simulink model "MALE_UAV_ENGINE"  (R2026a)
settings: Solver=ode45  StopTime=60
(part 1 of 2)
settings Model: Creator=stark  LastModifiedBy=stark
settings DataIOCC: OutputSaveName=simout

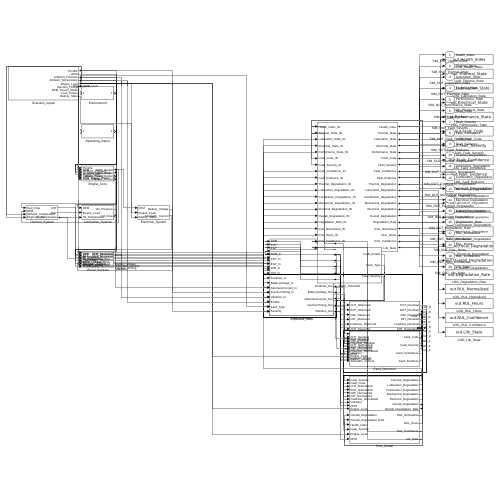
[thumbnail: Simulink's stored preview of the top-level diagram]
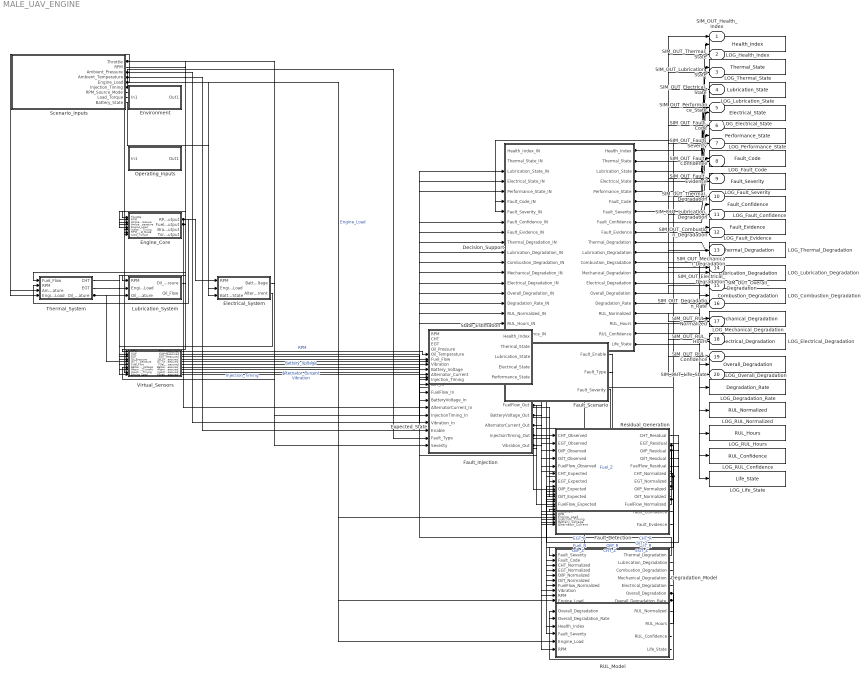
== system MALE_UAV_ENGINE ==
  Decision_Support : Subsystem
  Degradation_Model : Subsystem
  Electrical_System : Subsystem
  Engine_Core : Subsystem
  Environment : Subsystem
  Expected_State : Subsystem
  Fault_Detection : Subsystem
  Fault_Injection : Subsystem
  Fault_Scenario : Subsystem
  LOG_Combustion_Degradation : ToWorkspace  VariableName=Combustion_Degradation  SaveFormat=Timeseries  SampleTime=-1
  LOG_Degradation_Rate : ToWorkspace  VariableName=Degradation_Rate  SaveFormat=Timeseries  SampleTime=-1
  LOG_Electrical_Degradation : ToWorkspace  VariableName=Electrical_Degradation  SaveFormat=Timeseries  SampleTime=-1
  LOG_Electrical_State : ToWorkspace  VariableName=Electrical_State  SaveFormat=Timeseries  SampleTime=-1
  LOG_Fault_Code : ToWorkspace  VariableName=Fault_Code  SaveFormat=Timeseries  SampleTime=-1
  LOG_Fault_Confidence : ToWorkspace  VariableName=Fault_Confidence  SaveFormat=Timeseries  SampleTime=-1
  LOG_Fault_Evidence : ToWorkspace  VariableName=Fault_Evidence  SaveFormat=Timeseries  SampleTime=-1
  LOG_Fault_Severity : ToWorkspace  VariableName=Fault_Severity  SaveFormat=Timeseries  SampleTime=-1
  LOG_Health_Index : ToWorkspace  VariableName=Health_Index  SaveFormat=Timeseries  SampleTime=-1
  LOG_Life_State : ToWorkspace  VariableName=Life_State  SaveFormat=Timeseries  SampleTime=-1
  LOG_Lubrication_Degradation : ToWorkspace  VariableName=Lubrication_Degradation  SaveFormat=Timeseries  SampleTime=-1
  LOG_Lubrication_State : ToWorkspace  VariableName=Lubrication_State  SaveFormat=Timeseries  SampleTime=-1
  LOG_Mechanical_Degradation : ToWorkspace  VariableName=Mechanical_Degradation  SaveFormat=Timeseries  SampleTime=-1
  LOG_Overall_Degradation : ToWorkspace  VariableName=Overall_Degradation  SaveFormat=Timeseries  SampleTime=-1
  LOG_Performance_State : ToWorkspace  VariableName=Performance_State  SaveFormat=Timeseries  SampleTime=-1
  LOG_RUL_Confidence : ToWorkspace  VariableName=RUL_Confidence  SaveFormat=Timeseries  SampleTime=-1
  LOG_RUL_Hours : ToWorkspace  VariableName=RUL_Hours  SaveFormat=Timeseries  SampleTime=-1
  LOG_RUL_Normalized : ToWorkspace  VariableName=RUL_Normalized  SaveFormat=Timeseries  SampleTime=-1
  LOG_Thermal_Degradation : ToWorkspace  VariableName=Thermal_Degradation  SaveFormat=Timeseries  SampleTime=-1
  LOG_Thermal_State : ToWorkspace  VariableName=Thermal_State  SaveFormat=Timeseries  SampleTime=-1
  Lubrication_System : Subsystem
  Operating_Inputs : Subsystem
  RUL_Model : Subsystem
  Residual_Generation : Subsystem
  Scenario_Inputs : Subsystem
  State_Estimation : Subsystem
  Thermal_System : Subsystem
  Virtual_Sensors : Subsystem
  SIM_OUT_Health_Index : Outport  SignalName=Health_Index
  SIM_OUT_Thermal_State : Outport  Port=2  SignalName=Thermal_State
  SIM_OUT_Lubrication_State : Outport  Port=3  SignalName=Lubrication_State
  SIM_OUT_Electrical_State : Outport  Port=4  SignalName=Electrical_State
  SIM_OUT_Performance_State : Outport  Port=5  SignalName=Performance_State
  SIM_OUT_Fault_Code : Outport  Port=6  SignalName=Fault_Code
  SIM_OUT_Fault_Severity : Outport  Port=7  SignalName=Fault_Severity
  SIM_OUT_Fault_Confidence : Outport  Port=8  SignalName=Fault_Confidence
  SIM_OUT_Fault_Evidence : Outport  Port=9  SignalName=Fault_Evidence
  SIM_OUT_Thermal_Degradation : Outport  Port=10  SignalName=Thermal_Degradation
  SIM_OUT_Lubrication_Degradation : Outport  Port=11  SignalName=Lubrication_Degradation
  SIM_OUT_Combustion_Degradation : Outport  Port=12  SignalName=Combustion_Degradation
  SIM_OUT_Mechanical_Degradation : Outport  Port=13  SignalName=Mechanical_Degradation
  SIM_OUT_Electrical_Degradation : Outport  Port=14  SignalName=Electrical_Degradation
  SIM_OUT_Overall_Degradation : Outport  Port=15  SignalName=Overall_Degradation
  SIM_OUT_Degradation_Rate : Outport  Port=16  SignalName=Degradation_Rate
  SIM_OUT_RUL_Normalized : Outport  Port=17  SignalName=RUL_Normalized
  SIM_OUT_RUL_Hours : Outport  Port=18  SignalName=RUL_Hours
  SIM_OUT_RUL_Confidence : Outport  Port=19  SignalName=RUL_Confidence
  SIM_OUT_Life_State : Outport  Port=20  SignalName=Life_State
  wires:
  Scenario_Inputs/1(Throttle) -> Engine_Core/1(Throttle), Expected_State/6(Throttle)
  Scenario_Inputs/2(RPM) -> Engine_Core/2(RPM)
  Scenario_Inputs/3(Ambient_Pressure) -> Engine_Core/3(Ambient_Pressure), Expected_State/3(Ambient_Pressure)
  Scenario_Inputs/4(Ambient_Temperature) -> Engine_Core/4(Ambient_Temperature), Thermal_System/3(Ambient_Temperature), Expected_State/4(Ambient_Temperature)
  Scenario_Inputs/5(Engine_Load) -> Engine_Core/5(Engine_Load), Thermal_System/4(Engine_Load), Lubrication_System/2(Engine_Load), Electrical_System/2(Engine_Load), Virtual_Sensors/10(Engine_Load), Expected_State/2(Engine_Load), Fault_Detection/13(Engine_Load), Degradation_Model/10(Engine_Load), RUL_Model/5(Engine_Load)  "Engine_Load"
  Scenario_Inputs/6(Injection_Timing) -> Engine_Core/6(Injection_Timing), Virtual_Sensors/9(Injection_Timing), Expected_State/5(Injection_Timing)
  Scenario_Inputs/7(RPM_Source_Mode) -> Engine_Core/7(RPM_Source_Mode)
  Scenario_Inputs/8(Load_Torque) -> Engine_Core/8(Load_Torque)
  Engine_Core/2(Fuel_Flow_Output) -> Thermal_System/1(Fuel_Flow), Virtual_Sensors/6(Fuel_Flow)
  Engine_Core/1(RPM_Output) -> Thermal_System/2(RPM), Lubrication_System/1(RPM), Electrical_System/1(RPM), Virtual_Sensors/1(RPM), Expected_State/1(RPM)
  Thermal_System/3(Oil_Temperature) -> Lubrication_System/3(Oil_Temperature), Virtual_Sensors/5(Oil_Temperature)
  Scenario_Inputs/9(Battery_State) -> Electrical_System/3(Battery_State)
  Thermal_System/1(CHT) -> Virtual_Sensors/2(CHT)
  Thermal_System/2(EGT) -> Virtual_Sensors/3(EGT)
  Lubrication_System/1(Oil_Pressure) -> Virtual_Sensors/4(Oil_Pressure)
  Electrical_System/1(Battery_Voltage) -> Virtual_Sensors/7(Battery_Voltage)
  Electrical_System/2(Alternator_Current) -> Virtual_Sensors/8(Alternator_Current)
  Expected_State/1(Expected_CHT) -> Residual_Generation/6(CHT_Expected)
  Expected_State/2(Expected_EGT) -> Residual_Generation/7(EGT_Expected)
  Expected_State/3(Expected_Oil_Pressure) -> Residual_Generation/8(OilP_Expected)
  Expected_State/4(Expected_Oil_Temperature) -> Residual_Generation/9(OilT_Expected)
  Expected_State/5(Expected_Fuel_Flow) -> Residual_Generation/10(FuelFlow_Expected)
  Residual_Generation/1(CHT_Residual) -> Fault_Detection/1(CHT_Residual)  "CHT_R"
  Residual_Generation/2(EGT_Residual) -> Fault_Detection/2(EGT_Residual)  "EGT_R"
  Residual_Generation/3(OilP_Residual) -> Fault_Detection/3(OilP_Residual)  "OilP_R"
  Residual_Generation/4(OilT_Residual) -> Fault_Detection/4(OilT_Residual)  "OilT_R"
  Residual_Generation/5(FuelFlow_Residual) -> Fault_Detection/5(FuelFlow_Residual)  "Fuel_R"
  Residual_Generation/6(CHT_Normalized) -> Fault_Detection/6(CHT_Normalized), Degradation_Model/3(CHT_Normalized)  "CHT_Z"
  Residual_Generation/7(EGT_Normalized) -> Fault_Detection/7(EGT_Normalized), Degradation_Model/4(EGT_Normalized)  "EGT_Z"
  Residual_Generation/8(OilP_Normalized) -> Fault_Detection/8(OilP_Normalized), Degradation_Model/5(OilP_Normalized)  "OilP_Z"
  Residual_Generation/9(OilT_Normalized) -> Fault_Detection/9(OilT_Normalized), Degradation_Model/6(OilT_Normalized)  "OilT_Z"
  Residual_Generation/10(FuelFlow_Normalized) -> Fault_Detection/10(FuelFlow_Normalized), Degradation_Model/7(FuelFlow_Normalized)  "Fuel_Z"
  Fault_Detection/2(Fault_Severity) -> Degradation_Model/1(Fault_Severity), RUL_Model/4(Fault_Severity), Decision_Support/7(Fault_Severity_IN)
  Fault_Detection/1(Fault_Code) -> Degradation_Model/2(Fault_Code), Decision_Support/6(Fault_Code_IN)
  Degradation_Model/6(Overall_Degradation) -> RUL_Model/1(Overall_Degradation), Decision_Support/15(Overall_Degradation_IN)
  Degradation_Model/7(Overall_Degradation_Rate) -> RUL_Model/2(Overall_Degradation_Rate), Decision_Support/16(Degradation_Rate_IN)
  State_Estimation/1(Health_Index) -> RUL_Model/3(Health_Index), Decision_Support/1(Health_Index_IN)
  State_Estimation/2(Thermal_State) -> Decision_Support/2(Thermal_State_IN)
  State_Estimation/3(Lubrication_State) -> Decision_Support/3(Lubrication_State_IN)
  State_Estimation/4(Electrical_State) -> Decision_Support/4(Electrical_State_IN)
  State_Estimation/5(Performance_State) -> Decision_Support/5(Performance_State_IN)
  Fault_Detection/3(Fault_Confidence) -> Decision_Support/8(Fault_Confidence_IN)
  Fault_Detection/4(Fault_Evidence) -> Decision_Support/9(Fault_Evidence_IN)
  Degradation_Model/1(Thermal_Degradation) -> Decision_Support/10(Thermal_Degradation_IN)
  Degradation_Model/2(Lubrication_Degradation) -> Decision_Support/11(Lubrication_Degradation_IN)
  Degradation_Model/3(Combustion_Degradation) -> Decision_Support/12(Combustion_Degradation_IN)
  Degradation_Model/4(Mechanical_Degradation) -> Decision_Support/13(Mechanical_Degradation_IN)
  Degradation_Model/5(Electrical_Degradation) -> Decision_Support/14(Electrical_Degradation_IN)
  RUL_Model/1(RUL_Normalized) -> Decision_Support/17(RUL_Normalized_IN)
  RUL_Model/2(RUL_Hours) -> Decision_Support/18(RUL_Hours_IN)
  RUL_Model/3(RUL_Confidence) -> Decision_Support/19(RUL_Confidence_IN)
  RUL_Model/4(Life_State) -> Decision_Support/20(Life_State_IN)
  Decision_Support/1(Health_Index) -> LOG_Health_Index/1, SIM_OUT_Health_Index/1
  Decision_Support/2(Thermal_State) -> LOG_Thermal_State/1, SIM_OUT_Thermal_State/1
  Decision_Support/3(Lubrication_State) -> LOG_Lubrication_State/1, SIM_OUT_Lubrication_State/1
  Decision_Support/4(Electrical_State) -> LOG_Electrical_State/1, SIM_OUT_Electrical_State/1
  Decision_Support/5(Performance_State) -> LOG_Performance_State/1, SIM_OUT_Performance_State/1
  Decision_Support/6(Fault_Code) -> LOG_Fault_Code/1, SIM_OUT_Fault_Code/1
  Decision_Support/7(Fault_Severity) -> LOG_Fault_Severity/1, SIM_OUT_Fault_Severity/1
  Decision_Support/8(Fault_Confidence) -> LOG_Fault_Confidence/1, SIM_OUT_Fault_Confidence/1
  Decision_Support/9(Fault_Evidence) -> LOG_Fault_Evidence/1, SIM_OUT_Fault_Evidence/1
  Decision_Support/10(Thermal_Degradation) -> LOG_Thermal_Degradation/1, SIM_OUT_Thermal_Degradation/1
  Decision_Support/11(Lubrication_Degradation) -> LOG_Lubrication_Degradation/1, SIM_OUT_Lubrication_Degradation/1
  Decision_Support/12(Combustion_Degradation) -> LOG_Combustion_Degradation/1, SIM_OUT_Combustion_Degradation/1
  Decision_Support/13(Mechanical_Degradation) -> LOG_Mechanical_Degradation/1, SIM_OUT_Mechanical_Degradation/1
  Decision_Support/14(Electrical_Degradation) -> LOG_Electrical_Degradation/1, SIM_OUT_Electrical_Degradation/1
  Decision_Support/15(Overall_Degradation) -> LOG_Overall_Degradation/1, SIM_OUT_Overall_Degradation/1
  Decision_Support/16(Degradation_Rate) -> LOG_Degradation_Rate/1, SIM_OUT_Degradation_Rate/1
  Decision_Support/17(RUL_Normalized) -> LOG_RUL_Normalized/1, SIM_OUT_RUL_Normalized/1
  Decision_Support/18(RUL_Hours) -> LOG_RUL_Hours/1, SIM_OUT_RUL_Hours/1
  Decision_Support/19(RUL_Confidence) -> LOG_RUL_Confidence/1, SIM_OUT_RUL_Confidence/1
  Decision_Support/20(Life_State) -> LOG_Life_State/1, SIM_OUT_Life_State/1
  Fault_Scenario/1(Fault_Enable) -> Fault_Injection/11(Enable)
  Fault_Scenario/2(Fault_Type) -> Fault_Injection/12(Fault_Type)
  Fault_Scenario/3(Fault_Severity) -> Fault_Injection/13(Severity)
  Virtual_Sensors/1(RPM_Measured) -> Fault_Injection/1(RPM_In)  "RPM"
  Virtual_Sensors/2(CHT_Measured) -> Fault_Injection/2(CHT_In)
  Virtual_Sensors/3(EGT_Measured) -> Fault_Injection/3(EGT_In)
  Virtual_Sensors/4(Oil_Pressure_Measured) -> Fault_Injection/4(OilP_In)
  Virtual_Sensors/5(Oil_Temperature_Measured) -> Fault_Injection/5(OilT_In)
  Virtual_Sensors/6(Fuel_Flow_Measured) -> Fault_Injection/6(FuelFlow_In)
  Virtual_Sensors/7(Battery_Voltage_Measured) -> Fault_Injection/7(BatteryVoltage_In)  "Battery_Voltage"
  Virtual_Sensors/8(Alternator_Current_Measured) -> Fault_Injection/8(AlternatorCurrent_In)  "Alternator_Current"
  Virtual_Sensors/9(Injection_Timing_Measured) -> Fault_Injection/9(InjectionTiming_In)  "Injection_Timing"
  Virtual_Sensors/10(Vibration_Measured) -> Fault_Injection/10(Vibration_In)  "Vibration"
  Fault_Injection/1(RPM_Out) -> State_Estimation/1(RPM), Fault_Detection/12(RPM), Degradation_Model/9(RPM), RUL_Model/6(RPM)
  Fault_Injection/2(CHT_Out) -> State_Estimation/2(CHT), Residual_Generation/1(CHT_Observed)
  Fault_Injection/3(EGT_Out) -> State_Estimation/3(EGT), Residual_Generation/2(EGT_Observed)
  Fault_Injection/4(OilP_Out) -> State_Estimation/4(Oil_Pressure), Residual_Generation/3(OilP_Observed)
  Fault_Injection/5(OilT_Out) -> State_Estimation/5(Oil_Temperature), Residual_Generation/4(OilT_Observed)
  Fault_Injection/6(FuelFlow_Out) -> State_Estimation/6(Fuel_Flow), Residual_Generation/5(FuelFlow_Observed)
  Fault_Injection/7(BatteryVoltage_Out) -> State_Estimation/8(Battery_Voltage), Fault_Detection/15(Battery_Voltage)
  Fault_Injection/8(AlternatorCurrent_Out) -> State_Estimation/9(Alternator_Current), Fault_Detection/16(Alternator_Current)
  Fault_Injection/9(InjectionTiming_Out) -> State_Estimation/10(Injection_Timing), Fault_Detection/14(Injection_Timing)
  Fault_Injection/10(Vibration_Out) -> State_Estimation/7(Vibration), Fault_Detection/11(Vibration), Degradation_Model/8(Vibration)

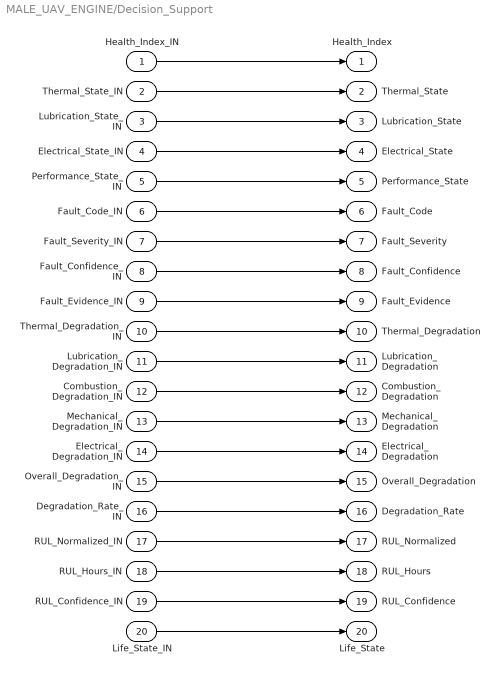
== system MALE_UAV_ENGINE/Decision_Support ==
  Health_Index_IN : Inport
  Thermal_State_IN : Inport  Port=2
  Lubrication_State_IN : Inport  Port=3
  Electrical_State_IN : Inport  Port=4
  Performance_State_IN : Inport  Port=5
  Fault_Code_IN : Inport  Port=6
  Fault_Severity_IN : Inport  Port=7
  Fault_Confidence_IN : Inport  Port=8
  Fault_Evidence_IN : Inport  Port=9
  Thermal_Degradation_IN : Inport  Port=10
  Lubrication_Degradation_IN : Inport  Port=11
  Combustion_Degradation_IN : Inport  Port=12
  Mechanical_Degradation_IN : Inport  Port=13
  Electrical_Degradation_IN : Inport  Port=14
  Overall_Degradation_IN : Inport  Port=15
  Degradation_Rate_IN : Inport  Port=16
  RUL_Normalized_IN : Inport  Port=17
  RUL_Hours_IN : Inport  Port=18
  RUL_Confidence_IN : Inport  Port=19
  Life_State_IN : Inport  Port=20
  Health_Index : Outport
  Thermal_State : Outport  Port=2
  Lubrication_State : Outport  Port=3
  Electrical_State : Outport  Port=4
  Performance_State : Outport  Port=5
  Fault_Code : Outport  Port=6
  Fault_Severity : Outport  Port=7
  Fault_Confidence : Outport  Port=8
  Fault_Evidence : Outport  Port=9
  Thermal_Degradation : Outport  Port=10
  Lubrication_Degradation : Outport  Port=11
  Combustion_Degradation : Outport  Port=12
  Mechanical_Degradation : Outport  Port=13
  Electrical_Degradation : Outport  Port=14
  Overall_Degradation : Outport  Port=15
  Degradation_Rate : Outport  Port=16
  RUL_Normalized : Outport  Port=17
  RUL_Hours : Outport  Port=18
  RUL_Confidence : Outport  Port=19
  Life_State : Outport  Port=20
  wires:
  ? -> ?
  Health_Index_IN/1 -> Health_Index/1
  Thermal_State_IN/1 -> Thermal_State/1
  Lubrication_State_IN/1 -> Lubrication_State/1
  Electrical_State_IN/1 -> Electrical_State/1
  Performance_State_IN/1 -> Performance_State/1
  Fault_Code_IN/1 -> Fault_Code/1
  Fault_Severity_IN/1 -> Fault_Severity/1
  Fault_Confidence_IN/1 -> Fault_Confidence/1
  Fault_Evidence_IN/1 -> Fault_Evidence/1
  Thermal_Degradation_IN/1 -> Thermal_Degradation/1
  Lubrication_Degradation_IN/1 -> Lubrication_Degradation/1
  Combustion_Degradation_IN/1 -> Combustion_Degradation/1
  Mechanical_Degradation_IN/1 -> Mechanical_Degradation/1
  Electrical_Degradation_IN/1 -> Electrical_Degradation/1
  Overall_Degradation_IN/1 -> Overall_Degradation/1
  Degradation_Rate_IN/1 -> Degradation_Rate/1
  RUL_Normalized_IN/1 -> RUL_Normalized/1
  RUL_Hours_IN/1 -> RUL_Hours/1
  RUL_Confidence_IN/1 -> RUL_Confidence/1
  Life_State_IN/1 -> Life_State/1

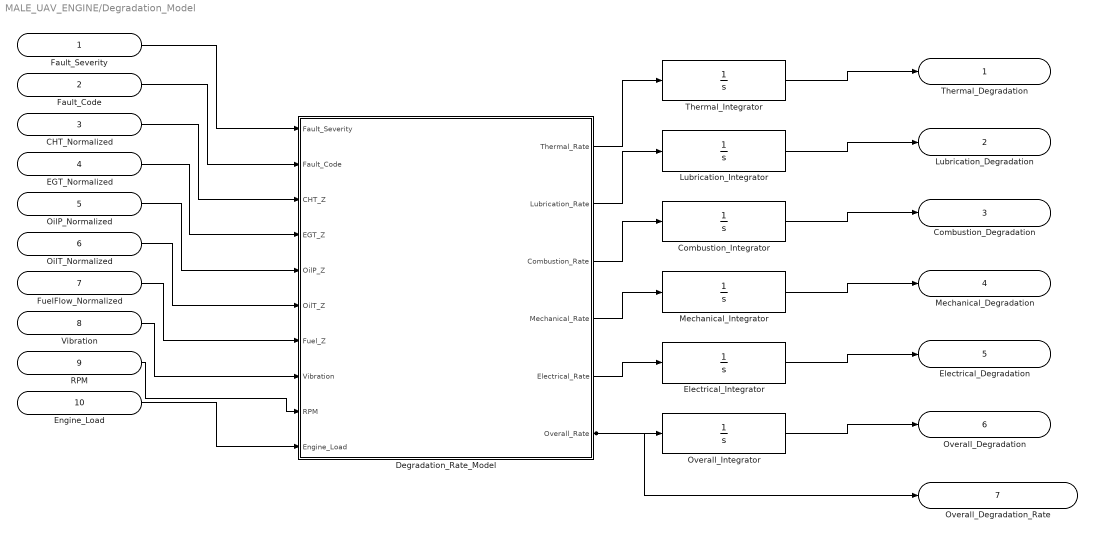
== system MALE_UAV_ENGINE/Degradation_Model ==
  Fault_Severity : Inport
  Fault_Code : Inport  Port=2
  CHT_Normalized : Inport  Port=3
  EGT_Normalized : Inport  Port=4
  OilP_Normalized : Inport  Port=5
  OilT_Normalized : Inport  Port=6
  FuelFlow_Normalized : Inport  Port=7
  Vibration : Inport  Port=8
  RPM : Inport  Port=9
  Engine_Load : Inport  Port=10
  Combustion_Integrator : Integrator  LimitOutput=on  UpperSaturationLimit=1  LowerSaturationLimit=0
  Degradation_Rate_Model : MATLAB Function  TreatAsAtomicUnit=on
  Electrical_Integrator : Integrator  LimitOutput=on  UpperSaturationLimit=1  LowerSaturationLimit=0
  Lubrication_Integrator : Integrator  LimitOutput=on  UpperSaturationLimit=1  LowerSaturationLimit=0
  Mechanical_Integrator : Integrator  LimitOutput=on  UpperSaturationLimit=1  LowerSaturationLimit=0
  Overall_Integrator : Integrator  LimitOutput=on  UpperSaturationLimit=1  LowerSaturationLimit=0
  Thermal_Integrator : Integrator  LimitOutput=on  UpperSaturationLimit=1  LowerSaturationLimit=0
  Thermal_Degradation : Outport
  Lubrication_Degradation : Outport  Port=2
  Combustion_Degradation : Outport  Port=3
  Mechanical_Degradation : Outport  Port=4
  Electrical_Degradation : Outport  Port=5
  Overall_Degradation : Outport  Port=6
  Overall_Degradation_Rate : Outport  Port=7
  wires:
  Fault_Severity/1 -> Degradation_Rate_Model/1(Fault_Severity)
  Fault_Code/1 -> Degradation_Rate_Model/2(Fault_Code)
  CHT_Normalized/1 -> Degradation_Rate_Model/3(CHT_Z)
  EGT_Normalized/1 -> Degradation_Rate_Model/4(EGT_Z)
  OilP_Normalized/1 -> Degradation_Rate_Model/5(OilP_Z)
  OilT_Normalized/1 -> Degradation_Rate_Model/6(OilT_Z)
  FuelFlow_Normalized/1 -> Degradation_Rate_Model/7(Fuel_Z)
  Vibration/1 -> Degradation_Rate_Model/8(Vibration)
  RPM/1 -> Degradation_Rate_Model/9(RPM)
  Engine_Load/1 -> Degradation_Rate_Model/10(Engine_Load)
  Degradation_Rate_Model/1(Thermal_Rate) -> Thermal_Integrator/1
  Degradation_Rate_Model/2(Lubrication_Rate) -> Lubrication_Integrator/1
  Degradation_Rate_Model/3(Combustion_Rate) -> Combustion_Integrator/1
  Degradation_Rate_Model/4(Mechanical_Rate) -> Mechanical_Integrator/1
  Degradation_Rate_Model/5(Electrical_Rate) -> Electrical_Integrator/1
  Degradation_Rate_Model/6(Overall_Rate) -> Overall_Integrator/1, Overall_Degradation_Rate/1
  Thermal_Integrator/1 -> Thermal_Degradation/1
  Lubrication_Integrator/1 -> Lubrication_Degradation/1
  Combustion_Integrator/1 -> Combustion_Degradation/1
  Mechanical_Integrator/1 -> Mechanical_Degradation/1
  Electrical_Integrator/1 -> Electrical_Degradation/1
  Overall_Integrator/1 -> Overall_Degradation/1

== system MALE_UAV_ENGINE/Electrical_System ==
  RPM : Inport
  Engine_Load : Inport  Port=2
  Battery_State : Inport  Port=3
  Battery_Voltage_Dynamics : TransferFcn  Denominator=[0.8 1]
  Electrical_Model : MATLAB Function  TreatAsAtomicUnit=on
  Battery_Voltage : Outport
  Alternator_Current : Outport  Port=2
  wires:
  RPM/1 -> Electrical_Model/1(RPM)
  Engine_Load/1 -> Electrical_Model/2(Engine_Load)
  Battery_State/1 -> Electrical_Model/3(Battery_State)
  Electrical_Model/1(Battery_Voltage) -> Battery_Voltage_Dynamics/1
  Battery_Voltage_Dynamics/1 -> Battery_Voltage/1
  Electrical_Model/2(Alternator_Current) -> Alternator_Current/1

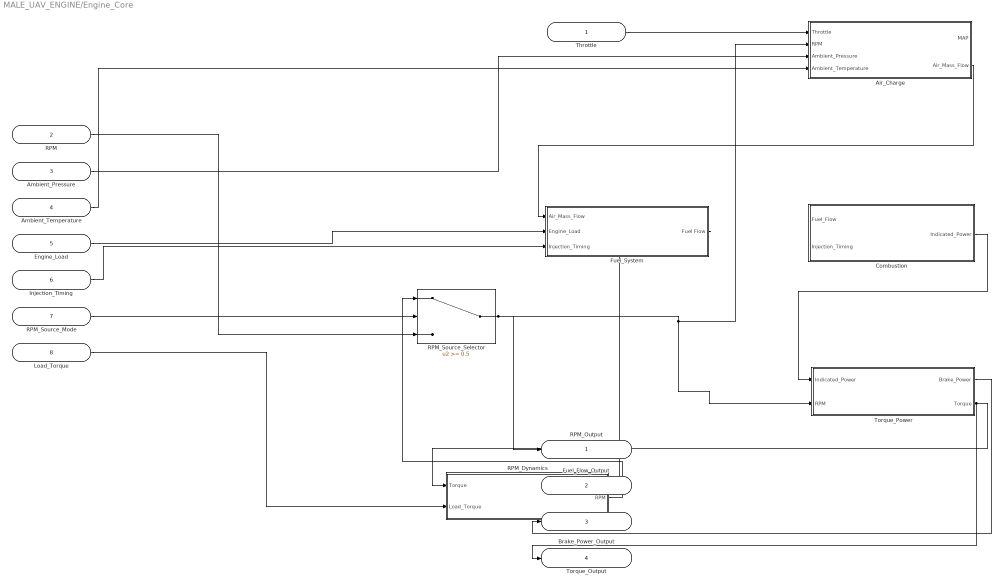
== system MALE_UAV_ENGINE/Engine_Core ==
  Throttle : Inport
  RPM : Inport  Port=2
  Ambient_Pressure : Inport  Port=3
  Ambient_Temperature : Inport  Port=4
  Engine_Load : Inport  Port=5
  Injection_Timing : Inport  Port=6
  RPM_Source_Mode : Inport  Port=7
  Load_Torque : Inport  Port=8
  Air_Charge : Subsystem
  Combustion : Subsystem
  Fuel_System : Subsystem
  RPM_Dynamics : Subsystem
  RPM_Source_Selector : Switch  Threshold=0.5  SaturateOnIntegerOverflow=off  InputSameDT=off
  Torque_Power : Subsystem
  RPM_Output : Outport
  Fuel_Flow_Output : Outport  Port=2
  Brake_Power_Output : Outport  Port=3
  Torque_Output : Outport  Port=4
  wires:
  Throttle/1 -> Air_Charge/1(Throttle)
  Ambient_Pressure/1 -> Air_Charge/3(Ambient_Pressure)
  Ambient_Temperature/1 -> Air_Charge/4(Ambient_Temperature)
  Engine_Load/1 -> Fuel_System/2(Engine_Load)
  Injection_Timing/1 -> Fuel_System/3(Injection_Timing)
  Air_Charge/2(Air_Mass_Flow) -> Fuel_System/1(Air_Mass_Flow)
  RPM_Dynamics/1(RPM) -> RPM_Source_Selector/1
  RPM_Source_Mode/1 -> RPM_Source_Selector/2
  RPM/1 -> RPM_Source_Selector/3
  RPM_Source_Selector/1 -> Torque_Power/2(RPM), Air_Charge/2(RPM), RPM_Output/1
  Combustion/1(Indicated_Power) -> Torque_Power/1(Indicated_Power)
  Torque_Power/2(Torque) -> RPM_Dynamics/1(Torque), Torque_Output/1
  Load_Torque/1 -> RPM_Dynamics/2(Load_Torque)
  Fuel_System/1(Fuel Flow) -> Fuel_Flow_Output/1
  Torque_Power/1(Brake_Power) -> Brake_Power_Output/1

== system MALE_UAV_ENGINE/Environment ==
  In1 : Inport
  Out1 : Outport
  wires:
  In1/1 -> Out1/1

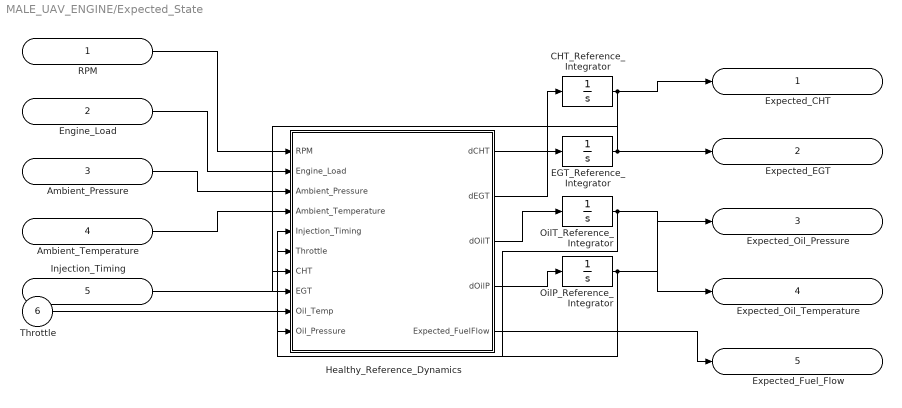
== system MALE_UAV_ENGINE/Expected_State ==
  RPM : Inport
  Engine_Load : Inport  Port=2
  Ambient_Pressure : Inport  Port=3
  Ambient_Temperature : Inport  Port=4
  Injection_Timing : Inport  Port=5
  Throttle : Inport  Port=6
  CHT_Reference_Integrator : Integrator  InitialCondition=373.15
  EGT_Reference_Integrator : Integrator  InitialCondition=873.15
  Healthy_Reference_Dynamics : MATLAB Function  TreatAsAtomicUnit=on
  OilP_Reference_Integrator : Integrator
  OilT_Reference_Integrator : Integrator  InitialCondition=363.15
  Expected_CHT : Outport
  Expected_EGT : Outport  Port=2
  Expected_Oil_Pressure : Outport  Port=3
  Expected_Oil_Temperature : Outport  Port=4
  Expected_Fuel_Flow : Outport  Port=5
  wires:
  RPM/1 -> Healthy_Reference_Dynamics/1(RPM)
  Engine_Load/1 -> Healthy_Reference_Dynamics/2(Engine_Load)
  Ambient_Pressure/1 -> Healthy_Reference_Dynamics/3(Ambient_Pressure)
  Ambient_Temperature/1 -> Healthy_Reference_Dynamics/4(Ambient_Temperature)
  Injection_Timing/1 -> Healthy_Reference_Dynamics/5(Injection_Timing)
  Throttle/1 -> Healthy_Reference_Dynamics/6(Throttle)
  CHT_Reference_Integrator/1 -> Healthy_Reference_Dynamics/7(CHT), Expected_CHT/1
  EGT_Reference_Integrator/1 -> Healthy_Reference_Dynamics/8(EGT), Expected_EGT/1
  OilT_Reference_Integrator/1 -> Healthy_Reference_Dynamics/9(Oil_Temp), Expected_Oil_Temperature/1
  OilP_Reference_Integrator/1 -> Healthy_Reference_Dynamics/10(Oil_Pressure), Expected_Oil_Pressure/1
  Healthy_Reference_Dynamics/1(dCHT) -> CHT_Reference_Integrator/1
  Healthy_Reference_Dynamics/2(dEGT) -> EGT_Reference_Integrator/1
  Healthy_Reference_Dynamics/3(dOilT) -> OilT_Reference_Integrator/1
  Healthy_Reference_Dynamics/4(dOilP) -> OilP_Reference_Integrator/1
  Healthy_Reference_Dynamics/5(Expected_FuelFlow) -> Expected_Fuel_Flow/1

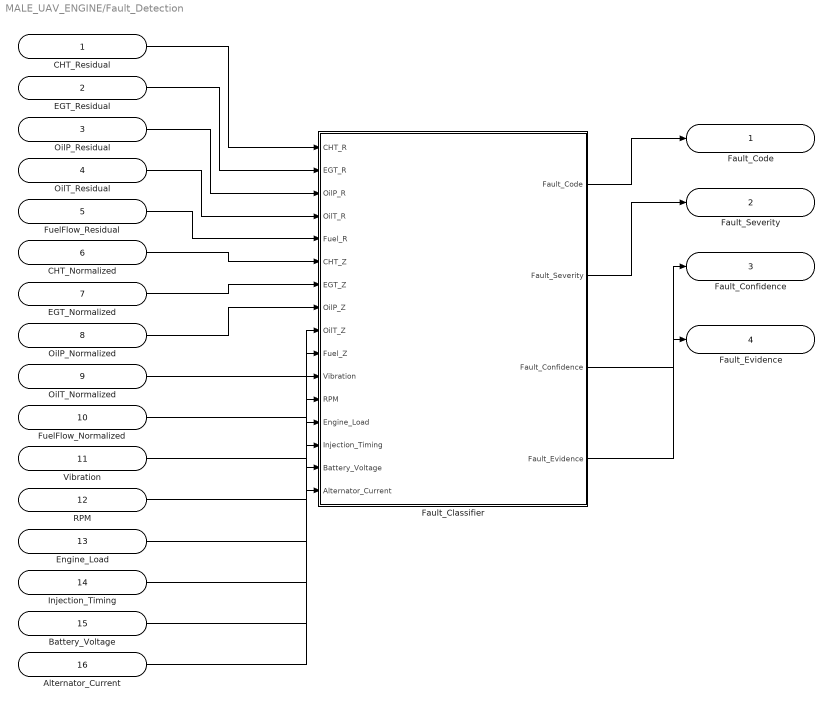
== system MALE_UAV_ENGINE/Fault_Detection ==
  CHT_Residual : Inport
  EGT_Residual : Inport  Port=2
  OilP_Residual : Inport  Port=3
  OilT_Residual : Inport  Port=4
  FuelFlow_Residual : Inport  Port=5
  CHT_Normalized : Inport  Port=6
  EGT_Normalized : Inport  Port=7
  OilP_Normalized : Inport  Port=8
  OilT_Normalized : Inport  Port=9
  FuelFlow_Normalized : Inport  Port=10
  Vibration : Inport  Port=11
  RPM : Inport  Port=12
  Engine_Load : Inport  Port=13
  Injection_Timing : Inport  Port=14
  Battery_Voltage : Inport  Port=15
  Alternator_Current : Inport  Port=16
  Fault_Classifier : MATLAB Function  TreatAsAtomicUnit=on
  Fault_Code : Outport
  Fault_Severity : Outport  Port=2
  Fault_Confidence : Outport  Port=3
  Fault_Evidence : Outport  Port=4
  wires:
  CHT_Residual/1 -> Fault_Classifier/1(CHT_R)
  EGT_Residual/1 -> Fault_Classifier/2(EGT_R)
  OilP_Residual/1 -> Fault_Classifier/3(OilP_R)
  OilT_Residual/1 -> Fault_Classifier/4(OilT_R)
  FuelFlow_Residual/1 -> Fault_Classifier/5(Fuel_R)
  CHT_Normalized/1 -> Fault_Classifier/6(CHT_Z)
  EGT_Normalized/1 -> Fault_Classifier/7(EGT_Z)
  OilP_Normalized/1 -> Fault_Classifier/8(OilP_Z)
  OilT_Normalized/1 -> Fault_Classifier/9(OilT_Z)
  FuelFlow_Normalized/1 -> Fault_Classifier/10(Fuel_Z)
  Vibration/1 -> Fault_Classifier/11(Vibration)
  RPM/1 -> Fault_Classifier/12(RPM)
  Engine_Load/1 -> Fault_Classifier/13(Engine_Load)
  Injection_Timing/1 -> Fault_Classifier/14(Injection_Timing)
  Battery_Voltage/1 -> Fault_Classifier/15(Battery_Voltage)
  Alternator_Current/1 -> Fault_Classifier/16(Alternator_Current)
  Fault_Classifier/1(Fault_Code) -> Fault_Code/1
  Fault_Classifier/2(Fault_Severity) -> Fault_Severity/1
  Fault_Classifier/3(Fault_Confidence) -> Fault_Confidence/1
  Fault_Classifier/4(Fault_Evidence) -> Fault_Evidence/1

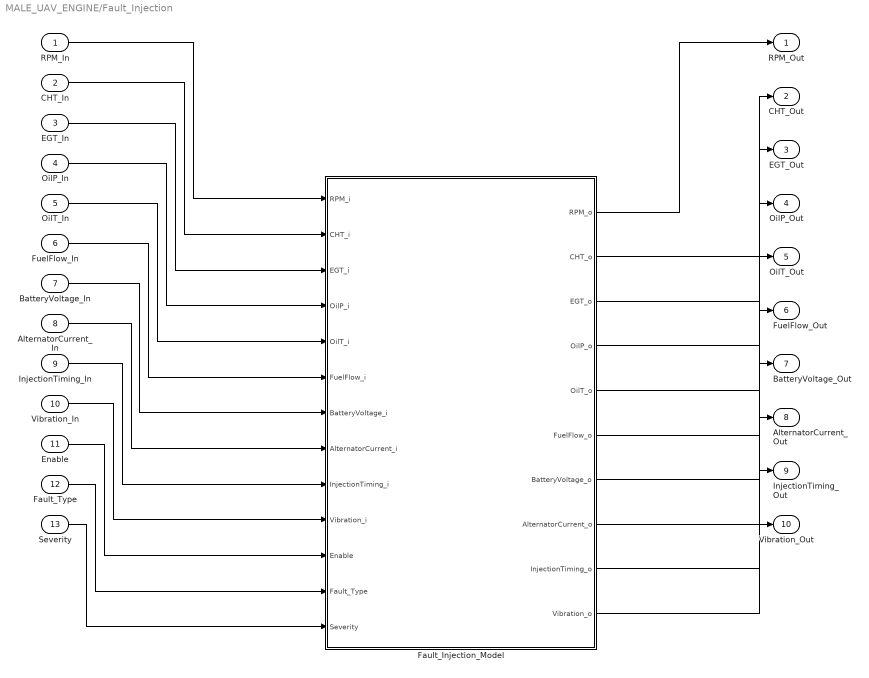
== system MALE_UAV_ENGINE/Fault_Injection ==
  RPM_In : Inport
  CHT_In : Inport  Port=2
  EGT_In : Inport  Port=3
  OilP_In : Inport  Port=4
  OilT_In : Inport  Port=5
  FuelFlow_In : Inport  Port=6
  BatteryVoltage_In : Inport  Port=7
  AlternatorCurrent_In : Inport  Port=8
  InjectionTiming_In : Inport  Port=9
  Vibration_In : Inport  Port=10
  Enable : Inport  Port=11
  Fault_Type : Inport  Port=12
  Severity : Inport  Port=13
  Fault_Injection_Model : MATLAB Function  TreatAsAtomicUnit=on
  RPM_Out : Outport
  CHT_Out : Outport  Port=2
  EGT_Out : Outport  Port=3
  OilP_Out : Outport  Port=4
  OilT_Out : Outport  Port=5
  FuelFlow_Out : Outport  Port=6
  BatteryVoltage_Out : Outport  Port=7
  AlternatorCurrent_Out : Outport  Port=8
  InjectionTiming_Out : Outport  Port=9
  Vibration_Out : Outport  Port=10
  wires:
  RPM_In/1 -> Fault_Injection_Model/1(RPM_i)
  CHT_In/1 -> Fault_Injection_Model/2(CHT_i)
  EGT_In/1 -> Fault_Injection_Model/3(EGT_i)
  OilP_In/1 -> Fault_Injection_Model/4(OilP_i)
  OilT_In/1 -> Fault_Injection_Model/5(OilT_i)
  FuelFlow_In/1 -> Fault_Injection_Model/6(FuelFlow_i)
  BatteryVoltage_In/1 -> Fault_Injection_Model/7(BatteryVoltage_i)
  AlternatorCurrent_In/1 -> Fault_Injection_Model/8(AlternatorCurrent_i)
  InjectionTiming_In/1 -> Fault_Injection_Model/9(InjectionTiming_i)
  Vibration_In/1 -> Fault_Injection_Model/10(Vibration_i)
  Enable/1 -> Fault_Injection_Model/11(Enable)
  Fault_Type/1 -> Fault_Injection_Model/12(Fault_Type)
  Severity/1 -> Fault_Injection_Model/13(Severity)
  Fault_Injection_Model/1(RPM_o) -> RPM_Out/1
  Fault_Injection_Model/2(CHT_o) -> CHT_Out/1
  Fault_Injection_Model/3(EGT_o) -> EGT_Out/1
  Fault_Injection_Model/4(OilP_o) -> OilP_Out/1
  Fault_Injection_Model/5(OilT_o) -> OilT_Out/1
  Fault_Injection_Model/6(FuelFlow_o) -> FuelFlow_Out/1
  Fault_Injection_Model/7(BatteryVoltage_o) -> BatteryVoltage_Out/1
  Fault_Injection_Model/8(AlternatorCurrent_o) -> AlternatorCurrent_Out/1
  Fault_Injection_Model/9(InjectionTiming_o) -> InjectionTiming_Out/1
  Fault_Injection_Model/10(Vibration_o) -> Vibration_Out/1

== system MALE_UAV_ENGINE/Fault_Scenario ==
  Enable : Constant  Value=0
  Severity : Constant  Value=0
  Type : Constant  Value=0
  Fault_Enable : Outport
  Fault_Type : Outport  Port=2
  Fault_Severity : Outport  Port=3
  wires:
  Enable/1 -> Fault_Enable/1
  Type/1 -> Fault_Type/1
  Severity/1 -> Fault_Severity/1

== system MALE_UAV_ENGINE/Lubrication_System ==
  RPM : Inport
  Engine_Load : Inport  Port=2
  Oil_Temperature : Inport  Port=3
  Lubrication_Model : MATLAB Function  TreatAsAtomicUnit=on
  Oil_Pressure_Dynamics : TransferFcn  Denominator=[0.5 1]
  Oil_Pressure : Outport
  Oil_Flow : Outport  Port=2
  wires:
  RPM/1 -> Lubrication_Model/1(RPM)
  Engine_Load/1 -> Lubrication_Model/2(Engine_Load)
  Oil_Temperature/1 -> Lubrication_Model/3(Oil_Temperature)
  Lubrication_Model/1(Target_Pressure) -> Oil_Pressure_Dynamics/1
  Oil_Pressure_Dynamics/1 -> Oil_Pressure/1
  Lubrication_Model/2(Oil_Flow) -> Oil_Flow/1

== system MALE_UAV_ENGINE/Operating_Inputs ==
  In1 : Inport
  Out1 : Outport
  wires:
  In1/1 -> Out1/1

== system MALE_UAV_ENGINE/RUL_Model ==
  Overall_Degradation : Inport
  Overall_Degradation_Rate : Inport  Port=2
  Health_Index : Inport  Port=3
  Fault_Severity : Inport  Port=4
  Engine_Load : Inport  Port=5
  RPM : Inport  Port=6
  RUL_Estimator : MATLAB Function  TreatAsAtomicUnit=on
  RUL_Normalized : Outport
  RUL_Hours : Outport  Port=2
  RUL_Confidence : Outport  Port=3
  Life_State : Outport  Port=4
  wires:
  ? -> ?
  Overall_Degradation/1 -> RUL_Estimator/1(Degradation)
  Overall_Degradation_Rate/1 -> RUL_Estimator/2(Degradation_Rate)
  Health_Index/1 -> RUL_Estimator/3(Health_Index)
  Fault_Severity/1 -> RUL_Estimator/4(Fault_Severity)
  Engine_Load/1 -> RUL_Estimator/5(Engine_Load)
  RPM/1 -> RUL_Estimator/6(RPM)
  RUL_Estimator/1(RUL_Normalized) -> RUL_Normalized/1
  RUL_Estimator/2(RUL_Hours) -> RUL_Hours/1
  RUL_Estimator/3(RUL_Confidence) -> RUL_Confidence/1
  RUL_Estimator/4(Life_State) -> Life_State/1

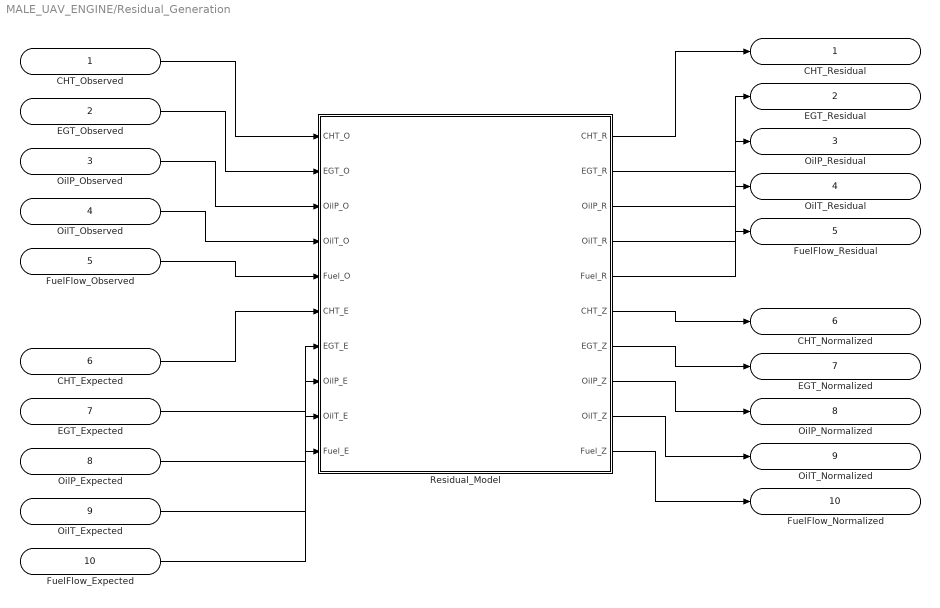
== system MALE_UAV_ENGINE/Residual_Generation ==
  CHT_Observed : Inport
  EGT_Observed : Inport  Port=2
  OilP_Observed : Inport  Port=3
  OilT_Observed : Inport  Port=4
  FuelFlow_Observed : Inport  Port=5
  CHT_Expected : Inport  Port=6
  EGT_Expected : Inport  Port=7
  OilP_Expected : Inport  Port=8
  OilT_Expected : Inport  Port=9
  FuelFlow_Expected : Inport  Port=10
  Residual_Model : MATLAB Function  TreatAsAtomicUnit=on
  CHT_Residual : Outport
  EGT_Residual : Outport  Port=2
  OilP_Residual : Outport  Port=3
  OilT_Residual : Outport  Port=4
  FuelFlow_Residual : Outport  Port=5
  CHT_Normalized : Outport  Port=6
  EGT_Normalized : Outport  Port=7
  OilP_Normalized : Outport  Port=8
  OilT_Normalized : Outport  Port=9
  FuelFlow_Normalized : Outport  Port=10
  wires:
  CHT_Observed/1 -> Residual_Model/1(CHT_O)
  EGT_Observed/1 -> Residual_Model/2(EGT_O)
  OilP_Observed/1 -> Residual_Model/3(OilP_O)
  OilT_Observed/1 -> Residual_Model/4(OilT_O)
  FuelFlow_Observed/1 -> Residual_Model/5(Fuel_O)
  CHT_Expected/1 -> Residual_Model/6(CHT_E)
  EGT_Expected/1 -> Residual_Model/7(EGT_E)
  OilP_Expected/1 -> Residual_Model/8(OilP_E)
  OilT_Expected/1 -> Residual_Model/9(OilT_E)
  FuelFlow_Expected/1 -> Residual_Model/10(Fuel_E)
  Residual_Model/1(CHT_R) -> CHT_Residual/1
  Residual_Model/2(EGT_R) -> EGT_Residual/1
  Residual_Model/3(OilP_R) -> OilP_Residual/1
  Residual_Model/4(OilT_R) -> OilT_Residual/1
  Residual_Model/5(Fuel_R) -> FuelFlow_Residual/1
  Residual_Model/6(CHT_Z) -> CHT_Normalized/1
  Residual_Model/7(EGT_Z) -> EGT_Normalized/1
  Residual_Model/8(OilP_Z) -> OilP_Normalized/1
  Residual_Model/9(OilT_Z) -> OilT_Normalized/1
  Residual_Model/10(Fuel_Z) -> FuelFlow_Normalized/1

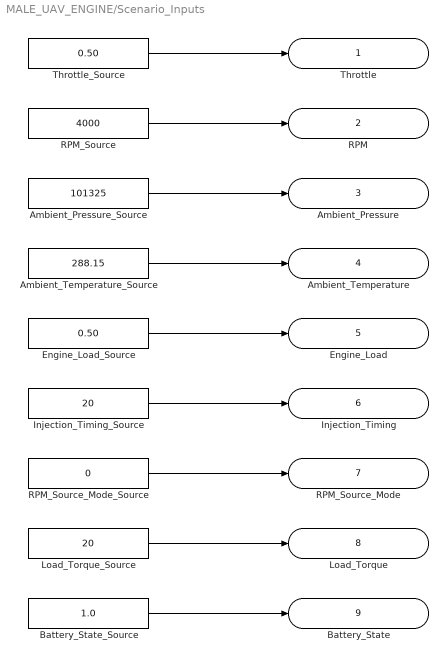
== system MALE_UAV_ENGINE/Scenario_Inputs ==
  Ambient_Pressure_Source : Constant  Value=101325
  Ambient_Temperature_Source : Constant  Value=288.15
  Battery_State_Source : Constant  Value=1.0
  Engine_Load_Source : Constant  Value=0.50
  Injection_Timing_Source : Constant  Value=20
  Load_Torque_Source : Constant  Value=20
  RPM_Source : Constant  Value=4000
  RPM_Source_Mode_Source : Constant  Value=0
  Throttle_Source : Constant  Value=0.50
  Throttle : Outport
  RPM : Outport  Port=2
  Ambient_Pressure : Outport  Port=3
  Ambient_Temperature : Outport  Port=4
  Engine_Load : Outport  Port=5
  Injection_Timing : Outport  Port=6
  RPM_Source_Mode : Outport  Port=7
  Load_Torque : Outport  Port=8
  Battery_State : Outport  Port=9
  wires:
  ? -> ?
  Throttle_Source/1 -> Throttle/1
  RPM_Source/1 -> RPM/1
  Ambient_Pressure_Source/1 -> Ambient_Pressure/1
  Ambient_Temperature_Source/1 -> Ambient_Temperature/1
  Engine_Load_Source/1 -> Engine_Load/1
  Injection_Timing_Source/1 -> Injection_Timing/1
  RPM_Source_Mode_Source/1 -> RPM_Source_Mode/1
  Load_Torque_Source/1 -> Load_Torque/1
  Battery_State_Source/1 -> Battery_State/1

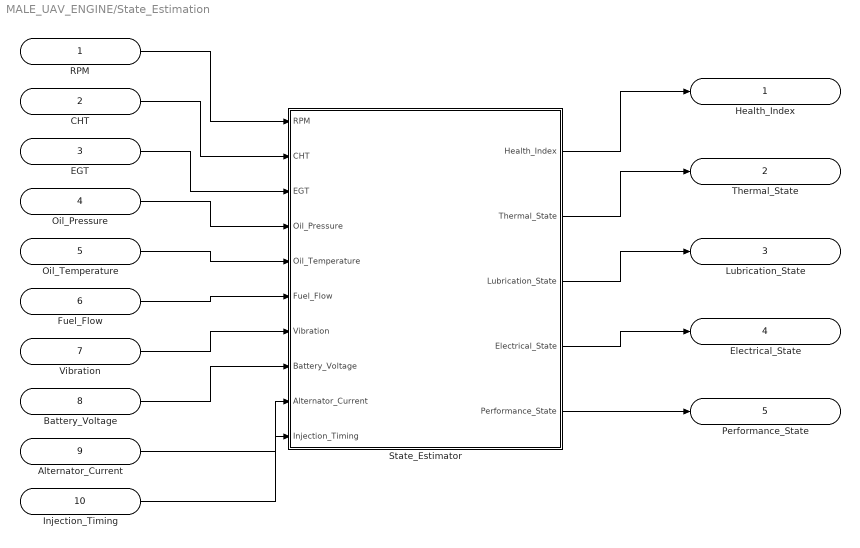
== system MALE_UAV_ENGINE/State_Estimation ==
  RPM : Inport
  CHT : Inport  Port=2
  EGT : Inport  Port=3
  Oil_Pressure : Inport  Port=4
  Oil_Temperature : Inport  Port=5
  Fuel_Flow : Inport  Port=6
  Vibration : Inport  Port=7
  Battery_Voltage : Inport  Port=8
  Alternator_Current : Inport  Port=9
  Injection_Timing : Inport  Port=10
  State_Estimator : MATLAB Function  TreatAsAtomicUnit=on
  Health_Index : Outport
  Thermal_State : Outport  Port=2
  Lubrication_State : Outport  Port=3
  Electrical_State : Outport  Port=4
  Performance_State : Outport  Port=5
  wires:
  RPM/1 -> State_Estimator/1(RPM)
  CHT/1 -> State_Estimator/2(CHT)
  EGT/1 -> State_Estimator/3(EGT)
  Oil_Pressure/1 -> State_Estimator/4(Oil_Pressure)
  Oil_Temperature/1 -> State_Estimator/5(Oil_Temperature)
  Fuel_Flow/1 -> State_Estimator/6(Fuel_Flow)
  Vibration/1 -> State_Estimator/7(Vibration)
  Battery_Voltage/1 -> State_Estimator/8(Battery_Voltage)
  Alternator_Current/1 -> State_Estimator/9(Alternator_Current)
  Injection_Timing/1 -> State_Estimator/10(Injection_Timing)
  State_Estimator/1(Health_Index) -> Health_Index/1
  State_Estimator/2(Thermal_State) -> Thermal_State/1
  State_Estimator/3(Lubrication_State) -> Lubrication_State/1
  State_Estimator/4(Electrical_State) -> Electrical_State/1
  State_Estimator/5(Performance_State) -> Performance_State/1

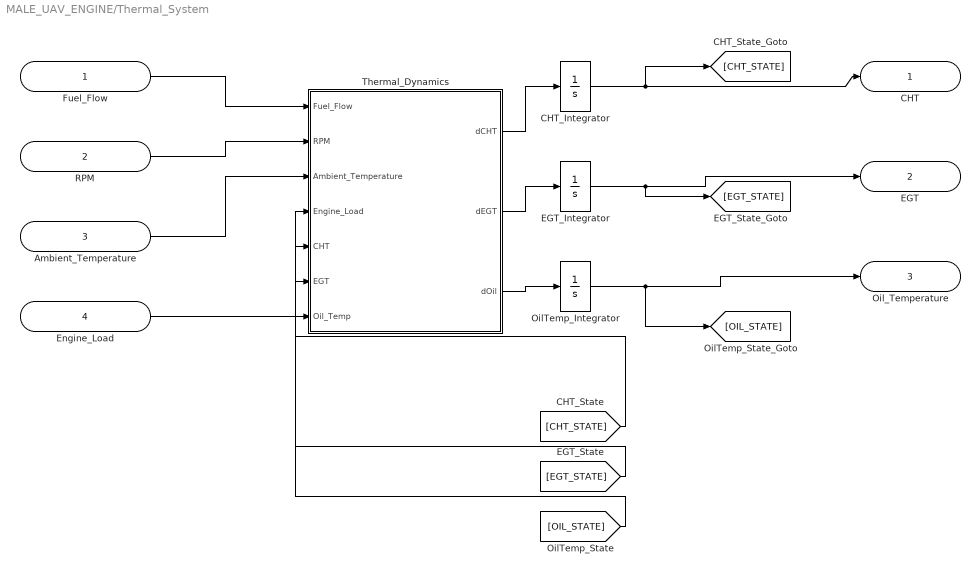
== system MALE_UAV_ENGINE/Thermal_System ==
  Fuel_Flow : Inport
  RPM : Inport  Port=2
  Ambient_Temperature : Inport  Port=3
  Engine_Load : Inport  Port=4
  CHT_Integrator : Integrator  InitialCondition=373.15
  EGT_Integrator : Integrator  InitialCondition=873.15
  OilTemp_Integrator : Integrator  InitialCondition=363.15
  Thermal_Dynamics : MATLAB Function  TreatAsAtomicUnit=on
  CHT : Outport
  EGT : Outport  Port=2
  Oil_Temperature : Outport  Port=3
  wires:
  Fuel_Flow/1 -> Thermal_Dynamics/1(Fuel_Flow)
  RPM/1 -> Thermal_Dynamics/2(RPM)
  Ambient_Temperature/1 -> Thermal_Dynamics/3(Ambient_Temperature)
  Engine_Load/1 -> Thermal_Dynamics/4(Engine_Load)
  [CHT_STATE] -> Thermal_Dynamics/5(CHT)
  [EGT_STATE] -> Thermal_Dynamics/6(EGT)
  [OIL_STATE] -> Thermal_Dynamics/7(Oil_Temp)
  Thermal_Dynamics/1(dCHT) -> CHT_Integrator/1
  Thermal_Dynamics/2(dEGT) -> EGT_Integrator/1
  Thermal_Dynamics/3(dOil) -> OilTemp_Integrator/1
  CHT_Integrator/1 -> CHT/1, [CHT_STATE]
  EGT_Integrator/1 -> EGT/1, [EGT_STATE]
  OilTemp_Integrator/1 -> Oil_Temperature/1, [OIL_STATE]

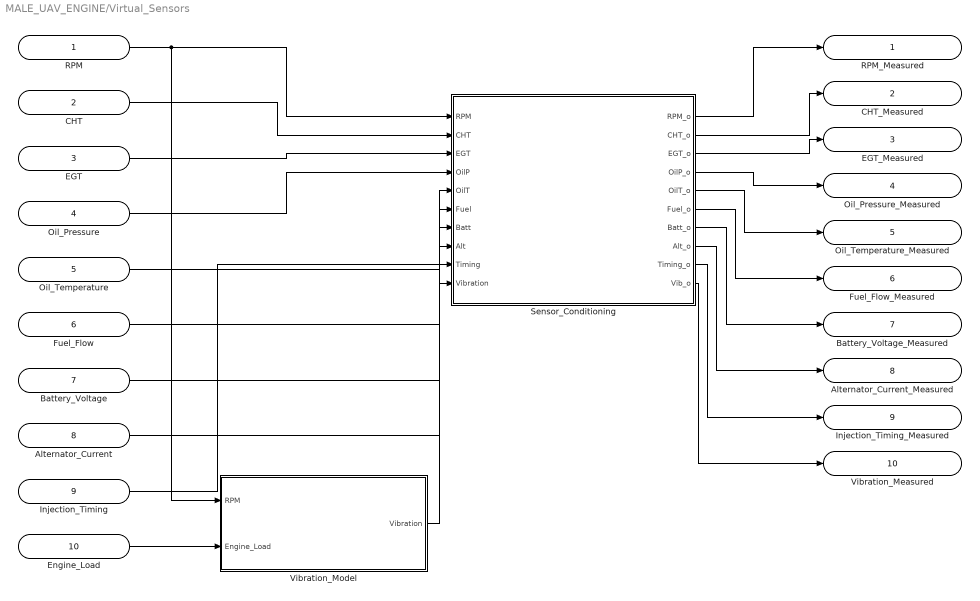
== system MALE_UAV_ENGINE/Virtual_Sensors ==
  RPM : Inport
  CHT : Inport  Port=2
  EGT : Inport  Port=3
  Oil_Pressure : Inport  Port=4
  Oil_Temperature : Inport  Port=5
  Fuel_Flow : Inport  Port=6
  Battery_Voltage : Inport  Port=7
  Alternator_Current : Inport  Port=8
  Injection_Timing : Inport  Port=9
  Engine_Load : Inport  Port=10
  Sensor_Conditioning : MATLAB Function  TreatAsAtomicUnit=on
  Vibration_Model : MATLAB Function  TreatAsAtomicUnit=on
  RPM_Measured : Outport
  CHT_Measured : Outport  Port=2
  EGT_Measured : Outport  Port=3
  Oil_Pressure_Measured : Outport  Port=4
  Oil_Temperature_Measured : Outport  Port=5
  Fuel_Flow_Measured : Outport  Port=6
  Battery_Voltage_Measured : Outport  Port=7
  Alternator_Current_Measured : Outport  Port=8
  Injection_Timing_Measured : Outport  Port=9
  Vibration_Measured : Outport  Port=10
  wires:
  RPM/1 -> Sensor_Conditioning/1(RPM), Vibration_Model/1(RPM)
  CHT/1 -> Sensor_Conditioning/2(CHT)
  EGT/1 -> Sensor_Conditioning/3(EGT)
  Oil_Pressure/1 -> Sensor_Conditioning/4(OilP)
  Oil_Temperature/1 -> Sensor_Conditioning/5(OilT)
  Fuel_Flow/1 -> Sensor_Conditioning/6(Fuel)
  Battery_Voltage/1 -> Sensor_Conditioning/7(Batt)
  Alternator_Current/1 -> Sensor_Conditioning/8(Alt)
  Injection_Timing/1 -> Sensor_Conditioning/9(Timing)
  Engine_Load/1 -> Vibration_Model/2(Engine_Load)
  Vibration_Model/1(Vibration) -> Sensor_Conditioning/10(Vibration)
  Sensor_Conditioning/1(RPM_o) -> RPM_Measured/1
  Sensor_Conditioning/2(CHT_o) -> CHT_Measured/1
  Sensor_Conditioning/3(EGT_o) -> EGT_Measured/1
  Sensor_Conditioning/4(OilP_o) -> Oil_Pressure_Measured/1
  Sensor_Conditioning/5(OilT_o) -> Oil_Temperature_Measured/1
  Sensor_Conditioning/6(Fuel_o) -> Fuel_Flow_Measured/1
  Sensor_Conditioning/7(Batt_o) -> Battery_Voltage_Measured/1
  Sensor_Conditioning/8(Alt_o) -> Alternator_Current_Measured/1
  Sensor_Conditioning/9(Timing_o) -> Injection_Timing_Measured/1
  Sensor_Conditioning/10(Vib_o) -> Vibration_Measured/1

== system MALE_UAV_ENGINE/Engine_Core/Air_Charge ==
  Throttle : Inport
  RPM : Inport  Port=2
  Ambient_Pressure : Inport  Port=3
  Ambient_Temperature : Inport  Port=4
  MATLAB Function : MATLAB Function  TreatAsAtomicUnit=on
  MAP : Outport
  Air_Mass_Flow : Outport  Port=2
  wires:
  Throttle/1 -> MATLAB Function/1(Throttle)
  RPM/1 -> MATLAB Function/2(RPM)
  Ambient_Pressure/1 -> MATLAB Function/3(Ambient_Pressure)
  Ambient_Temperature/1 -> MATLAB Function/4(Ambient_Temperature)
  MATLAB Function/1(MAP) -> MAP/1
  MATLAB Function/2(Air_Mass_Flow) -> Air_Mass_Flow/1

== system MALE_UAV_ENGINE/Engine_Core/Combustion ==
  Fuel_Flow : Inport
  Injection_Timing : Inport  Port=2
  Combustion_Model : MATLAB Function  TreatAsAtomicUnit=on
  Indicated_Power : Outport
  wires:
  Fuel_Flow/1 -> Combustion_Model/1(Fuel_Flow)
  Injection_Timing/1 -> Combustion_Model/2(Injection_Timing)
  Combustion_Model/1(Indicated_Power) -> Indicated_Power/1

== system MALE_UAV_ENGINE/Engine_Core/Fuel_System ==
  Air_Mass_Flow : Inport
  Engine_Load : Inport  Port=2
  Injection_Timing : Inport  Port=3
  MATLAB Function : MATLAB Function  TreatAsAtomicUnit=on
  Fuel Flow : Outport
  wires:
  Injection_Timing/1 -> MATLAB Function/3(Injection_Timing)
  Engine_Load/1 -> MATLAB Function/2(Engine_Load)
  MATLAB Function/1(Fuel_Flow) -> Fuel Flow/1
  Air_Mass_Flow/1 -> MATLAB Function/1(Air_Mass_Flow)

== system MALE_UAV_ENGINE/Engine_Core/RPM_Dynamics ==
  Torque : Inport
  Load_Torque : Inport  Port=2
  Angular_Velocity : Integrator  InitialCondition=146.607657167524
  Inverse_Inertia : Gain  Gain=10
  Net_Torque : Sum  Inputs=+-
  RPM_Limiter : Saturate  UpperLimit=5800  LowerLimit=0
  RadPerSec_to_RPM : Gain  Gain=9.54929658551372
  RPM : Outport
  wires:
  Torque/1 -> Net_Torque/1
  Load_Torque/1 -> Net_Torque/2
  Net_Torque/1 -> Inverse_Inertia/1
  Inverse_Inertia/1 -> Angular_Velocity/1
  Angular_Velocity/1 -> RadPerSec_to_RPM/1
  RadPerSec_to_RPM/1 -> RPM_Limiter/1
  RPM_Limiter/1 -> RPM/1

== system MALE_UAV_ENGINE/Engine_Core/Torque_Power ==
  Indicated_Power : Inport
  RPM : Inport  Port=2
  Torque_Power_Model : MATLAB Function  TreatAsAtomicUnit=on
  Brake_Power : Outport
  Torque : Outport  Port=2
  wires:
  Indicated_Power/1 -> Torque_Power_Model/1(Indicated_Power)
  RPM/1 -> Torque_Power_Model/2(RPM)
  Torque_Power_Model/1(Brake_Power) -> Brake_Power/1
  Torque_Power_Model/2(Torque) -> Torque/1

== matlab function MALE_UAV_ENGINE/Virtual_Sensors/Vibration_Model ==
  data: RPM input; Vibration output; Engine_Load input
function Vibration = fcn(RPM, Engine_Load)
% SIH26 Digital Twin
% Virtual vibration sensor V1

    RPM = max(0, RPM);
    Engine_Load = max(0, min(1, Engine_Load));

    base_vibration = 0.25;
    rotational_component = 0.00015 * RPM;
    load_component = 1.5 * Engine_Load;

    Vibration = ...
        base_vibration ...
        + rotational_component ...
        + load_component;

end

== matlab function MALE_UAV_ENGINE/Virtual_Sensors/Sensor_Conditioning ==
  data: RPM input; RPM_o output; CHT input; EGT input; OilP input; OilT input; Fuel input; Batt input; Alt input; Timing input; Vibration input; CHT_o output; EGT_o output; OilP_o output; OilT_o output; Fuel_o output; Batt_o output; Alt_o output; Timing_o output; Vib_o output
function [RPM_o, CHT_o, EGT_o, OilP_o, OilT_o, Fuel_o, Batt_o, Alt_o, Timing_o, Vib_o] = ...
fcn(RPM, CHT, EGT, OilP, OilT, Fuel, Batt, Alt, Timing, Vibration)
% SIH26 Digital Twin
% Standardized Virtual Sensor Conditioning
% V1

    %% Sensor bias parameters
    rpm_bias = 0;
    cht_bias = 0;
    egt_bias = 0;
    oilp_bias = 0;
    oilt_bias = 0;
    fuel_bias = 0;
    batt_bias = 0;
    alt_bias = 0;
    timing_bias = 0;
    vibration_bias = 0;

    %% Conditioned telemetry
    RPM_o = RPM + rpm_bias;
    CHT_o = CHT + cht_bias;
    EGT_o = EGT + egt_bias;
    OilP_o = OilP + oilp_bias;
    OilT_o = OilT + oilt_bias;
    Fuel_o = max(0, Fuel + fuel_bias);
    Batt_o = Batt + batt_bias;
    Alt_o = max(0, Alt + alt_bias);
    Timing_o = Timing + timing_bias;
    Vib_o = max(0, Vibration + vibration_bias);

end

== matlab function MALE_UAV_ENGINE/State_Estimation/State_Estimator ==
  data: RPM input; Health_Index output; CHT input; EGT input; Oil_Pressure input; Oil_Temperature input; Fuel_Flow input; Vibration input; Battery_Voltage input; Alternator_Current input; Injection_Timing input; Thermal_State output; Lubrication_State output; Electrical_State output; Performance_State output
function [Health_Index, Thermal_State, Lubrication_State, Electrical_State, Performance_State] = ...
fcn(RPM, CHT, EGT, Oil_Pressure, Oil_Temperature, Fuel_Flow, Vibration, Battery_Voltage, Alternator_Current, Injection_Timing)
% SIH26 Digital Twin
% State Estimation Layer V1
%
% Converts standardized telemetry into normalized
% engine state indicators.
%
% Outputs are normalized approximately to [0,1],
% where 1 represents healthy nominal operation.

    %% Nominal reference values
    RPM_nom = 4000;
    CHT_nom = 390;
    EGT_nom = 1050;
    OilP_nom = 250000;
    OilT_nom = 380;
    Fuel_nom = 0.0015;
    Vibration_nom = 1.2;
    Battery_nom = 14;
    Alternator_nom = 20;
    Timing_nom = 20;

    %% RPM state
    rpm_score = 1 - abs(RPM - RPM_nom) / RPM_nom;
    rpm_score = max(0, min(1, rpm_score));

    %% Thermal state
    cht_score = 1 - max(0, CHT - CHT_nom) / 80;
    egt_score = 1 - max(0, EGT - EGT_nom) / 300;
    oil_temp_score = 1 - max(0, Oil_Temperature - OilT_nom) / 100;

    Thermal_State = mean([cht_score egt_score oil_temp_score]);
    Thermal_State = max(0, min(1, Thermal_State));

    %% Lubrication state
    oil_pressure_score = min(1, Oil_Pressure / OilP_nom);
    oil_temperature_lube_score = 1 - max(0, Oil_Temperature - OilT_nom) / 100;

    Lubrication_State = mean([oil_pressure_score oil_temperature_lube_score]);
    Lubrication_State = max(0, min(1, Lubrication_State));

    %% Electrical state
    battery_score = min(1, Battery_Voltage / Battery_nom);
    alternator_score = min(1, Alternator_Current / Alternator_nom);

    Electrical_State = mean([battery_score alternator_score]);
    Electrical_State = max(0, min(1, Electrical_State));

    %% Performance state
    vibration_score = 1 - max(0, Vibration - Vibration_nom) / 3;
    timing_score = 1 - abs(Injection_Timing - Timing_nom) / 20;
    fuel_score = 1 - abs(Fuel_Flow - Fuel_nom) / max(Fuel_nom, 1e-6);

    vibration_score = max(0, min(1, vibration_score));
    timing_score = max(0, min(1, timing_score));
    fuel_score = max(0, min(1, fuel_score));

    Performance_State = mean([rpm_score vibration_score timing_score fuel_score]);
    Performance_State = max(0, min(1, Performance_State));

    %% Overall health
    Health_Index = mean([ ...
        Thermal_State ...
        Lubrication_State ...
        Electrical_State ...
        Performance_State ]);

    Health_Index = max(0, min(1, Health_Index));

end

== matlab function MALE_UAV_ENGINE/Expected_State/Healthy_Reference_Dynamics ==
  data: RPM input; dCHT output; Engine_Load input; Ambient_Pressure input; Ambient_Temperature input; Injection_Timing input; Throttle input; CHT input; EGT input; Oil_Temp input; Oil_Pressure input; dEGT output; dOilT output; dOilP output; Expected_FuelFlow output
function [dCHT,dEGT,dOilT,dOilP,Expected_FuelFlow] = fcn(RPM,Engine_Load,Ambient_Pressure,Ambient_Temperature,Injection_Timing,Throttle,CHT,EGT,Oil_Temp,Oil_Pressure)
% SIH26 Digital Twin
% Independent healthy dynamic reference model V1

    RPM = max(0,RPM);
    Engine_Load = max(0,min(1,Engine_Load));
    Ambient_Temperature = max(200,Ambient_Temperature);
    Ambient_Pressure = max(20000,Ambient_Pressure);
    Throttle = max(0,min(1,Throttle));

    %% Air charge
    R_air = 287.05;
    VE = 0.80;
    displacement = 1.352e-3;
    MAP = Ambient_Pressure * Throttle;
    Air_Mass_Flow = ...
        (MAP * displacement / ...
        (R_air * Ambient_Temperature)) ...
        * (RPM / 120) * VE;

    %% Fuel system
    AFR = 14.7;
    combustion_efficiency = 0.98;
    timing_error = Injection_Timing - 20;
    timing_efficiency = ...
        max(0,1 - 0.001 * timing_error^2);
    Expected_FuelFlow = ...
        (Air_Mass_Flow / AFR) ...
        * combustion_efficiency ...
        * timing_efficiency ...
        * Engine_Load;

    %% Thermal dynamics
    LHV = 43e6;
    Fuel_Power = Expected_FuelFlow * LHV;
    Q_CHT_in = 0.08 * Fuel_Power;
    Q_EGT_in = 0.30 * Fuel_Power;
    Q_Oil_in = 0.04 * Fuel_Power;

    CHT_cooling = ...
        (20 + 0.015 * RPM) ...
        * max(CHT - Ambient_Temperature,0);

    EGT_cooling = ...
        (8 + 0.004 * RPM) ...
        * max(EGT - Ambient_Temperature,0);

    Oil_cooling = ...
        (12 + 0.008 * RPM) ...
        * max(Oil_Temp - Ambient_Temperature,0);

    CHT_capacity = 20000;
    EGT_capacity = 5000;
    Oil_capacity = 15000;

    dCHT = (Q_CHT_in - CHT_cooling) / CHT_capacity;
    dEGT = (Q_EGT_in - EGT_cooling) / EGT_capacity;
    dOilT = (Q_Oil_in - Oil_cooling) / Oil_capacity;

    %% Lubrication dynamics
    reference_temperature = 373.15;
    reference_viscosity = 0.020;
    viscosity = reference_viscosity * ...
        exp(-0.025 * (Oil_Temp-reference_temperature));
    viscosity = max(viscosity,0.002);

    pump_factor = RPM / 5800;
    load_factor = 0.30 + 0.70 * Engine_Load;
    base_pressure = 500000;
    pressure_gain = 2500000 * pump_factor * load_factor;
    viscosity_factor = reference_viscosity / viscosity;
    Target_Pressure = base_pressure + ...
        pressure_gain * viscosity_factor;

    Target_Pressure = max(0,Target_Pressure);
    dOilP = (Target_Pressure - Oil_Pressure) / 0.5;

end

== matlab function MALE_UAV_ENGINE/Residual_Generation/Residual_Model ==
  data: CHT_O input; CHT_R output; EGT_O input; OilP_O input; OilT_O input; Fuel_O input; CHT_E input; EGT_E input; OilP_E input; OilT_E input; Fuel_E input; EGT_R output; OilP_R output; OilT_R output; Fuel_R output; CHT_Z output; EGT_Z output; OilP_Z output; OilT_Z output; Fuel_Z output
function [CHT_R, EGT_R, OilP_R, OilT_R, Fuel_R, CHT_Z, EGT_Z, OilP_Z, OilT_Z, Fuel_Z] = ...
fcn(CHT_O, EGT_O, OilP_O, OilT_O, Fuel_O, CHT_E, EGT_E, OilP_E, OilT_E, Fuel_E)
% SIH26 Digital Twin
% Residual Generation Layer V1
%
% Residual = observed - expected.
% Z-score-like normalized residuals provide
% scale-independent diagnostic features.

    %% Absolute residuals
    CHT_R = CHT_O - CHT_E;
    EGT_R = EGT_O - EGT_E;
    OilP_R = OilP_O - OilP_E;
    OilT_R = OilT_O - OilT_E;
    Fuel_R = Fuel_O - Fuel_E;

    %% Representative residual scales
    CHT_sigma = 10;
    EGT_sigma = 30;
    OilP_sigma = 25000;
    OilT_sigma = 10;
    Fuel_sigma = 0.00015;

    %% Normalized residuals
    CHT_Z = CHT_R / CHT_sigma;
    EGT_Z = EGT_R / EGT_sigma;
    OilP_Z = OilP_R / OilP_sigma;
    OilT_Z = OilT_R / OilT_sigma;
    Fuel_Z = Fuel_R / Fuel_sigma;

end
